simulink model "Sim6"  (R2019a)
settings: Solver=VariableStepAuto  StartTime=0.0  StopTime=10.0  RelTol=1e-3
settings Model: Creator=fbleo  LastModifiedBy=fbleo

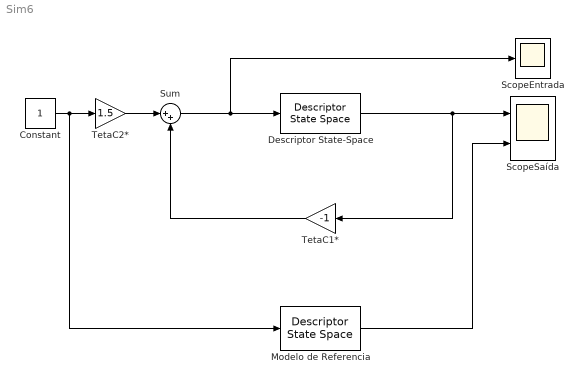
== system Sim6 ==
  "    TetaC1*" : Gain  Gain=-1
  Constant : Constant
  Descriptor State-Space : DescriptorStateSpace  A=-1  B=2  D=0  InitialCondition=0.5
  Modelo de Referencia : DescriptorStateSpace  A=-3  B=3  D=0  InitialCondition=0
  ScopeEntrada : Scope
  ScopeSaída : Scope  NumInputPorts=2
  Sum : Sum  Inputs=|++
  TetaC2* : Gain  Gain=1.5
  wires:
  Descriptor State-Space/1 -> "    TetaC1*"/1, ScopeSaída/1
  Sum/1 -> ScopeEntrada/1, Descriptor State-Space/1
  "    TetaC1*"/1 -> Sum/2
  TetaC2*/1 -> Sum/1
  Constant/1 -> Modelo de Referencia/1, TetaC2*/1
  Modelo de Referencia/1 -> ScopeSaída/2
